simulink model "TST_AdvancedStateflowLoops2"  (Simulink 7.4)
settings: Solver=FixedStepDiscrete  StartTime=0.0  StopTime=10.0  FixedStep=0.02  RelTol=1e-3
settings Model: Creator=kharthforeign  LastModifiedBy=kharthforeign  BufferReuse=off
settings DataIOCC: SaveOutput=off  SignalLogging=off  SaveTime=off
settings OptimizationCC: BlockReduction=off  ConditionallyExecuteInputs=off  OptimizeBlockIOStorage=off  BufferReuse=off  ExpressionFolding=off  LocalBlockOutputs=off  InitFltsAndDblsToZero=on

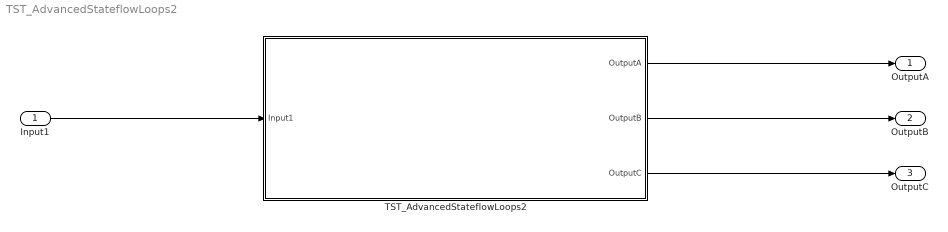
== system TST_AdvancedStateflowLoops2 ==
  Input1 : Inport  DataType=uint32  OutDataType=fixdt(1, 16)  OutScaling=2^0  OutDataTypeStr=uint32  BusOutputAsStruct=on
  TST_AdvancedStateflowLoops2 : Subsystem  TreatAsAtomicUnit=on
  OutputA : Outport  PortDimensions=1  DataType=double  OutDataType=fixdt(1, 16)  OutScaling=2^0  OutDataTypeStr=double
  OutputB : Outport  Port=2  PortDimensions=1  DataType=double  OutDataType=Enum: DIL_VmmGsFcsCommandsMessage_LatApModeCmd  OutDataTypeStr=double
  OutputC : Outport  Port=3  PortDimensions=1  DataType=double  OutDataType=fixdt(1, 16)  OutScaling=2^0  OutDataTypeStr=double
  wires:
  Input1/1 -> TST_AdvancedStateflowLoops2/1(Input1)
  TST_AdvancedStateflowLoops2/1(OutputA) -> OutputA/1
  TST_AdvancedStateflowLoops2/2(OutputB) -> OutputB/1
  TST_AdvancedStateflowLoops2/3(OutputC) -> OutputC/1

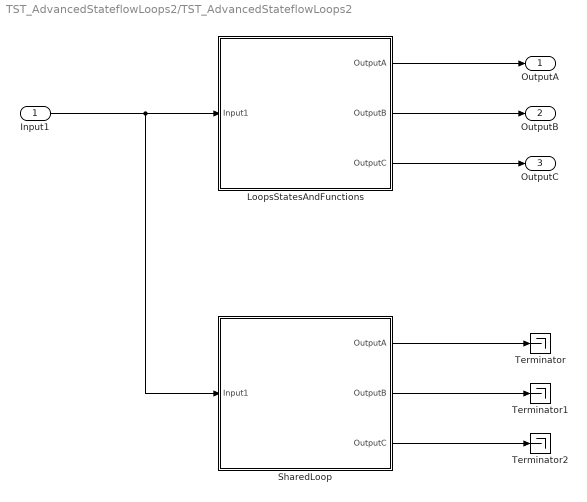
== system TST_AdvancedStateflowLoops2/TST_AdvancedStateflowLoops2 ==
  Input1 : Inport  DataType=uint32  OutDataType=fixdt(1, 16)  OutScaling=2^0  OutDataTypeStr=uint32  BusOutputAsStruct=on
  LoopsStatesAndFunctions : Stateflow chart
  SharedLoop : Stateflow chart
  Terminator : Terminator
  Terminator1 : Terminator
  Terminator2 : Terminator
  OutputA : Outport  PortDimensions=1  DataType=double  OutDataType=fixdt(1, 16)  OutScaling=2^0  OutDataTypeStr=double
  OutputB : Outport  Port=2  PortDimensions=1  DataType=double  OutDataType=Enum: DIL_VmmGsFcsCommandsMessage_LatApModeCmd  OutDataTypeStr=double
  OutputC : Outport  Port=3  PortDimensions=1  DataType=double  OutDataType=fixdt(1, 16)  OutScaling=2^0  OutDataTypeStr=double
  wires:
  LoopsStatesAndFunctions/1(OutputA) -> OutputA/1
  LoopsStatesAndFunctions/2(OutputB) -> OutputB/1
  LoopsStatesAndFunctions/3(OutputC) -> OutputC/1
  Input1/1 -> LoopsStatesAndFunctions/1(Input1), SharedLoop/1(Input1)
  SharedLoop/1(OutputA) -> Terminator/1
  SharedLoop/2(OutputB) -> Terminator1/1
  SharedLoop/3(OutputC) -> Terminator2/1

== stateflow chart TST_AdvancedStateflowLoops2/LoopsStatesAndFunctions ==
  state Ping
  state Pong
    state PongSubA
    state PongSubB
    note: demonstrate a loop inside a state
    (default) -> (junction 11)
    (junction 11) -> (junction 11) [order 1] : [C]{OutputC = 5.0;}
    (junction 11) -> PongSubA [order 2]
    PongSubA -> PongSubB : [Iterate(uint32(3))]
    PongSubB -> PongSubA : [Iterate(uint32(4))]
  state x = Iterate(b) [function]
    note: demonstrate a loop instide a function
    (default) -> (junction 14) : {Count = uint32(0);}
    (junction 14) -> (junction 15) [order 1] : [Count < b]...
        | {Count += uint32(1);}
    (junction 15) -> (junction 14) : {OutputC = ...
        | OutputC * OutputC;}
    (junction 14) -> (junction 16) [order 2] : {x = true;}
  note: demonstrate a loop between states
  (default) -> Ping
  Ping -> Pong [order 1] : [A]{OutputA = 2.0;}
  Ping -> (junction 12) [order 2]
  (junction 12) -> (junction 13) [order 1] : [B]{OutputB = 3.0;}
  (junction 13) -> (junction 12) : {OutputB += 1.0;}
  (junction 12) -> Pong [order 2]
  data: Count temporary uint32; b function_input uint32; x function_output boolean; Input1 input uint32; OutputA output double =1; OutputB output double =2; OutputC output double =3; Local local uint32 =0; A local boolean; B local boolean; C local boolean

== stateflow chart TST_AdvancedStateflowLoops2/SharedLoop ==
  state StateA
  state StateB
  state StateC
  note: demonstrate a flowgraph-loop on a joined path
      | with two different sources
  (default) -> StateA
  (junction 50) -> (junction 51) [order 1] : [B]
  (junction 51) -> (junction 52)
  (junction 52) -> (junction 50) : {OutputB += 2.0}
  (junction 49) -> (junction 50) : [A]
  (junction 50) -> StateC [order 2] : /{OutputC = 7.0}
  StateA -> (junction 49) [order 2]
  StateA -> StateB [order 1] : [Input1 > 5]
  StateB -> (junction 49) : [Input1 < 5]
  data: Input1 input uint32; OutputA output double =1; OutputB output double =2; OutputC output double =3; Local local uint32 =0; A local boolean; B local boolean; C local boolean; D local boolean
